simulink model "TwoSinusoidsCloseTogether"  (R2017b)
settings: Solver=FixedStepDiscrete  StartTime=0.0  StopTime=inf  RelTol=1e-3
libraries: dspsrcs4 x3
settings Model: Creator=rlosada  LastModifiedBy=rlosada
settings SolverCC: AutoInsertRateTranBlk=on
settings DataIOCC: LimitDataPoints=on  SaveOutput=off  SignalLogging=off  SaveTime=off
settings OptimizationCC: LifeSpan=inf  SimCompilerOptimization=on
settings DebuggingCC: AlgebraicLoopMsg=error  SingleTaskRateTransMsg=error  AllowSymbolicDim=off  SFUnexpectedBacktrackingDiag=warning  SFNoUnconditionalDefaultTransitionDiag=warning  SFExecutionAtInitializationDiag=none
settings CodeAppCC: StateflowObjectComments=on
settings GRTTargetCC: TargetLangStandard=C89/C90 (ANSI)  GeneratePreprocessorConditionals=Disable all
settings ConfigComp: CovMetricSettings=dw  CovHtmlReporting=on  CovSaveCumulativeToWorkspaceVar=on  CovSaveSingleToWorkspaceVar=on  CovExternalEMLEnable=off  CovSFcnEnable=off

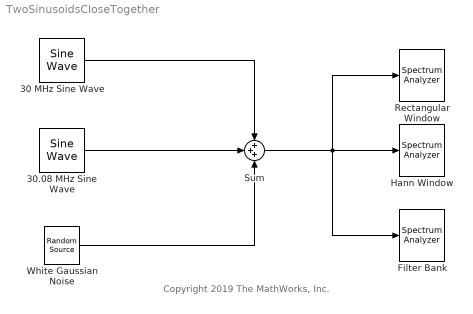
== system TwoSinusoidsCloseTogether ==
  note: Copyright 2019 The MathWorks, Inc.
  30 MHz Sine Wave : dspsrcs4/Sine Wave  Amplitude=1  Frequency=30e6  Phase=0  SampleMode=Discrete  OutComplex=Real  CompMethod=Trigonometric fcn  TableSize=Speed  SampleTime=1/100e6  SamplesPerFrame=2500  ResetState=Restart at time zero  OutputFrames=off  dataType=double  wordLen=16  udDataType=sfix(16)  fracBitsMode=Best precision  numFracBits=15  OutDataTypeStr=double  LastOutDataTypeStr=double
  30.08 MHz Sine Wave : dspsrcs4/Sine Wave  Amplitude=1  Frequency=30.08e6  Phase=0  SampleMode=Discrete  OutComplex=Real  CompMethod=Trigonometric fcn  TableSize=Speed  SampleTime=1/100e6  SamplesPerFrame=2500  ResetState=Restart at time zero  OutputFrames=off  dataType=double  wordLen=16  udDataType=sfix(16)  fracBitsMode=Best precision  numFracBits=15  OutDataTypeStr=double  LastOutDataTypeStr=double
  Filter Bank : SpectrumAnalyzer
  Hann Window : SpectrumAnalyzer
  Rectangular Window : SpectrumAnalyzer
  Sum : Sum  Inputs=+++
  White Gaussian Noise : dspsrcs4/Random Source  SrcType=Gaussian  NormMethod=Ziggurat  CltLength=12  MinVal=0  MaxVal=1  MeanVal=0  VarVal=0.1111111111111111  RepMode=Not repeatable  rawSeed=1  IsInherit=off  SampMode=Discrete  SampTime=1/100e6  SampFrame=2500  DataType=Double  OutComplex=Real  OutputFrames=off
  wires:
  30.08 MHz Sine Wave/1 -> Sum/2
  30 MHz Sine Wave/1 -> Sum/1
  Sum/1 -> Filter Bank/1, Hann Window/1, Rectangular Window/1
  White Gaussian Noise/1 -> Sum/3
